simulink model "wwb_2"  (Simulink 6.0)
settings: Solver=ode45  StartTime=0.0  StopTime=10.0  RelTol=1e-3
libraries: simulink x1
settings Model: LastModifiedBy=paul

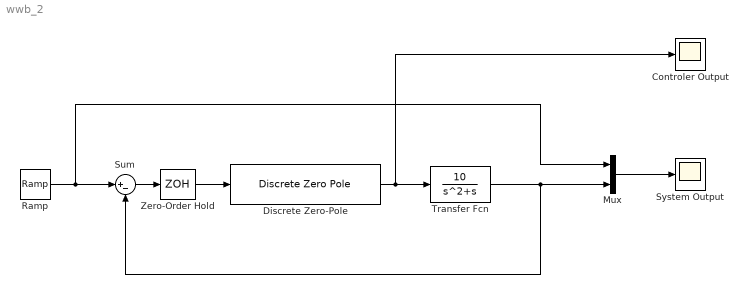
== system wwb_2 ==
  Controler Output : Scope
      settings: YMin=-500  YMax=500
  Discrete Zero-Pole : DiscreteZeroPole  Zeros=[0.3679 0.5859]  Poles=[1 -0.592]  Gain=0.383
  Mux : Mux  Inputs=2
  Ramp : simulink/Sources/Ramp  slope=1  start=0  X0=0
  Sum : Sum  Inputs=|+-
  System Output : Scope
      settings: YMin=-2  YMax=12
  Transfer Fcn : TransferFcn  Numerator=[10]  Denominator=[1 1 0]
  Zero-Order Hold : ZeroOrderHold
  wires:
  Zero-Order Hold/1 -> Discrete Zero-Pole/1
  Sum/1 -> Zero-Order Hold/1
  Discrete Zero-Pole/1 -> Transfer Fcn/1, Controler Output/1
  Ramp/1 -> Sum/1, Mux/1
  Mux/1 -> System Output/1
  Transfer Fcn/1 -> Sum/2, Mux/2
